simulink model "ModelTest"  (R2019b)
settings: Solver=ode4  StartTime=0.0  StopTime=10  FixedStep=0.001  RelTol=1e-3
settings Model: Creator=B210b  LastModifiedBy=B210b

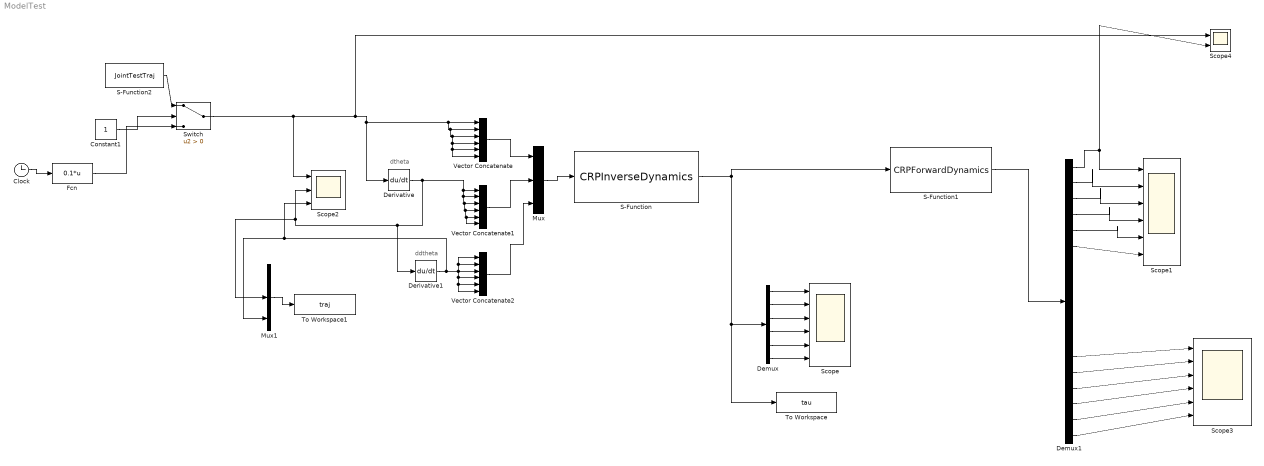
== system ModelTest ==
  note: ddtheta
  note: dtheta
  Clock : Clock
  Constant1 : Constant
  Demux : Demux  Outputs=6
  Demux1 : Demux  Outputs=18
  Derivative : Derivative  CoefficientInTFapproximation=0
  Derivative1 : Derivative  CoefficientInTFapproximation=0
  Fcn : Fcn  Expr=0.1*u
  Mux : Mux  Inputs=3
  Mux1 : Mux  Inputs=3
  S-Function : S-Function  FunctionName=CRPInverseDynamics  SFunctionDeploymentMode=off  EnableBusSupport=off
  S-Function1 : S-Function  FunctionName=CRPForwardDynamics  SFunctionDeploymentMode=off  EnableBusSupport=off
  S-Function2 : S-Function  FunctionName=JointTestTraj  SFunctionDeploymentMode=off  EnableBusSupport=off
  Scope : Scope  NumInputPorts=6
  Scope1 : Scope  NumInputPorts=6
  Scope2 : Scope  NumInputPorts=3
  Scope3 : Scope  NumInputPorts=6
  Scope4 : Scope  NumInputPorts=2
  Switch : Switch  Criteria=u2 > Threshold
  To Workspace : ToWorkspace  VariableName=tau  SaveFormat=Timeseries  SampleTime=-1
  To Workspace1 : ToWorkspace  VariableName=traj  SaveFormat=Timeseries  SampleTime=-1
  Vector Concatenate : Concatenate  NumInputs=6
  Vector Concatenate1 : Concatenate  NumInputs=6
  Vector Concatenate2 : Concatenate  NumInputs=6
  wires:
  Mux/1 -> S-Function/1
  Demux/1 -> Scope/1
  Demux/2 -> Scope/2
  Demux/3 -> Scope/3
  Demux/4 -> Scope/4
  Demux/5 -> Scope/5
  Demux/6 -> Scope/6
  S-Function/1 -> To Workspace/1, Demux/1, S-Function1/1
  Vector Concatenate/1 -> Mux/1
  Vector Concatenate1/1 -> Mux/2
  Vector Concatenate2/1 -> Mux/3
  Derivative/1 -> Vector Concatenate1/6, Vector Concatenate1/5, Vector Concatenate1/4, Vector Concatenate1/3, Vector Concatenate1/2, Vector Concatenate1/1, Mux1/2, Scope2/2, Derivative1/1
  Derivative1/1 -> Mux1/3, Scope2/3, Vector Concatenate2/6, Vector Concatenate2/5, Vector Concatenate2/4, Vector Concatenate2/3, Vector Concatenate2/2, Vector Concatenate2/1
  S-Function1/1 -> Demux1/1
  Demux1/1 -> Scope4/2, Scope1/1
  Demux1/2 -> Scope1/2
  Demux1/3 -> Scope1/3
  Demux1/4 -> Scope1/4
  Demux1/5 -> Scope1/5
  Demux1/6 -> Scope1/6
  Mux1/1 -> To Workspace1/1
  Demux1/13 -> Scope3/1
  Demux1/14 -> Scope3/2
  Demux1/15 -> Scope3/3
  Demux1/16 -> Scope3/4
  Demux1/17 -> Scope3/5
  Demux1/18 -> Scope3/6
  Fcn/1 -> Switch/3
  S-Function2/1 -> Switch/1
  Switch/1 -> Scope2/1, Scope4/1, Derivative/1, Vector Concatenate/6, Vector Concatenate/5, Vector Concatenate/4, Vector Concatenate/3, Vector Concatenate/2, Vector Concatenate/1
  Constant1/1 -> Switch/2
  Clock/1 -> Fcn/1
